simulink model "linear_model"  (R2021a)
settings: Solver=VariableStepAuto  StartTime=0.0  StopTime=30  RelTol=1e-3
values from neighbouring files (symbols this model uses):
  K_omega_z_int = get_K_value(K_omega_z_calc, q_calc, mach_calc(i), H_calc)    [short_period.m]
  K_theta_int = get_K_value(K_theta_calc, q_calc, mach_calc(i), H_calc)    [short_period.m]
libraries: cstblocks x6
settings Model: Creator=lalapopa  LastModifiedBy=lalapopa

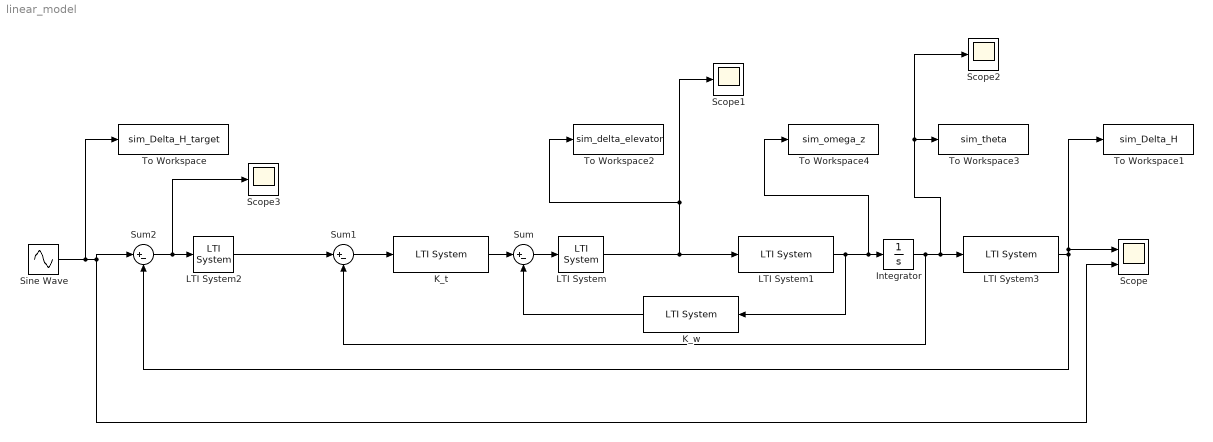
== system linear_model ==
  Integrator : Integrator
  K_t : cstblocks/LTI System  sys=-K_theta_int  IC=[]
  K_w : cstblocks/LTI System  sys=-K_omega_z_int  IC=[]
  LTI System : cstblocks/LTI System  sys=W_p  IC=[]
  LTI System1 : cstblocks/LTI System  sys=d_w_d_v  IC=[]
  LTI System2 : cstblocks/LTI System  sys=i_H  IC=[]
  LTI System3 : cstblocks/LTI System  sys=W_H_theta  IC=[]
  Scope : Scope  NumInputPorts=2
  Scope1 : Scope
  Scope2 : Scope
  Scope3 : Scope
  Sine Wave : Sin  SampleTime=0
  Sum : Sum  Inputs=|+-
  Sum1 : Sum  Inputs=|+-
  Sum2 : Sum  Inputs=|+-
  To Workspace : ToWorkspace  VariableName=sim_Delta_H_target  SaveFormat=Timeseries  SampleTime=-1
      settings: Decimation=3  Save2DSignal=2-D array (concatenate along first dimension)
  To Workspace1 : ToWorkspace  VariableName=sim_Delta_H  SaveFormat=Timeseries  SampleTime=-1
  To Workspace2 : ToWorkspace  VariableName=sim_delta_elevator  SaveFormat=Timeseries  SampleTime=-1
  To Workspace3 : ToWorkspace  VariableName=sim_theta  SaveFormat=Timeseries  SampleTime=-1
  To Workspace4 : ToWorkspace  VariableName=sim_omega_z  SaveFormat=Timeseries  SampleTime=-1
  wires:
  LTI System1/1 -> K_w/1, To Workspace4/1, Integrator/1
  Sum/1 -> LTI System/1
  K_w/1 -> Sum/2
  LTI System3/1 -> Scope/1, To Workspace1/1, Sum2/2
  LTI System2/1 -> Sum1/1
  Sum1/1 -> K_t/1
  LTI System/1 -> Scope1/1, To Workspace2/1, LTI System1/1
  Sum2/1 -> Scope3/1, LTI System2/1
  Integrator/1 -> Scope2/1, To Workspace3/1, LTI System3/1, Sum1/2
  K_t/1 -> Sum/1
  Sine Wave/1 -> To Workspace/1, Scope/2, Sum2/1
